simulink model "AltitudeHold_ModernControlH"  (R2024b)
settings: Solver=VariableStepAuto  StartTime=0.0  StopTime=500  RelTol=1e-3
values from neighbouring files (symbols this model uses):
  sysLong = ss(A,B,C,D,'statename',states,'inputname',inputs,'outputname',outputs)    [AltitudeHold_ModernControl.m]    (also in PitchAttitudeHold_ModernControl.m = ss(A,B,C,D))
undefined symbols (not defined in the file or in its folder): Kh
settings Model: Creator=wangdi  LastModifiedBy=wangdi

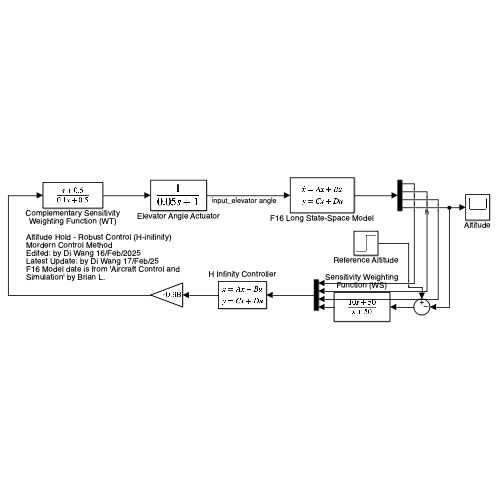
[thumbnail: Simulink's stored preview of the top-level diagram]
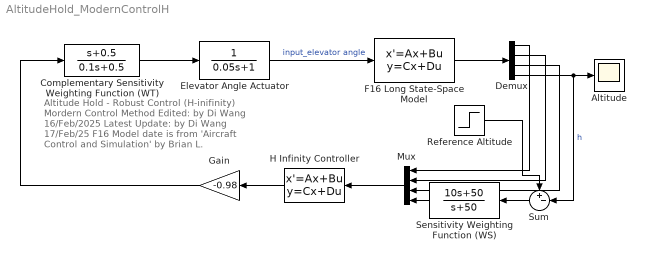
== system AltitudeHold_ModernControlH ==
  note: Altitude Hold - Robust Control (H-inifinity)
      | Mordern Control Method
      | Edited: by Di Wang 16/Feb/2025
      | Latest Update: by Di Wang 17/Feb/25
      | F16 Model date is from 'Aircraft Control and Simulation' by Brian L.
  Altitude : Scope
  Complementary Sensitivity Weighting Function (WT) : TransferFcn  Numerator=[1 0.5]  Denominator=[0.1 0.5]
  Demux : Demux
  Elevator Angle Actuator : TransferFcn  Denominator=[0.05 1]
  F16 Long State-Space Model : StateSpace  A=sysLong.A  B=sysLong.B  C=sysLong.C  D=sysLong.D  InitialCondition=0
  Gain : Gain  Gain=-0.98
  H Infinity Controller : StateSpace  A=Kh.A  B=Kh.B  C=Kh.C  D=Kh.D  InitialCondition=0
  Mux : Mux
  Reference Altitude : Step  After=1000  SampleTime=0
  Sensitivity Weighting Function (WS) : TransferFcn  Numerator=[10 50]  Denominator=[1 50]
  Sum : Sum  Inputs=+-|
  wires:
  Elevator Angle Actuator/1 -> F16 Long State-Space Model/1  "input_elevator angle"
  F16 Long State-Space Model/1 -> Demux/1
  Demux/4 -> Sum/2, Altitude/1  "h"
  Demux/3 -> Mux/3
  Demux/2 -> Mux/2
  Demux/1 -> Mux/1
  H Infinity Controller/1 -> Gain/1
  Reference Altitude/1 -> Sum/1
  Complementary Sensitivity Weighting Function (WT)/1 -> Elevator Angle Actuator/1
  Sum/1 -> Sensitivity Weighting Function (WS)/1
  Mux/1 -> H Infinity Controller/1
  Sensitivity Weighting Function (WS)/1 -> Mux/4
  Gain/1 -> Complementary Sensitivity Weighting Function (WT)/1
